simulink model "elevator"  (R2026a)
settings: Solver=VariableStepAuto  StopTime=inf
(part 2 of 2)

== stateflow chart elevator/Chart ==
  state moveup
    entry:
    movedirection=1;
    doorstatus=0;
  state movedown
    entry:
    movedirection=-1;
    doorstatus=0;
  state idle
    entry:
    movedirection=0;
    doorstatus=0;
    during:
    if(floor1==1)
    requestedfloor=0;
    end
    if(floor2==1)
    requestedfloor=1;
    end
    if(floor3==1)
    requestedfloor=2;
    end
  state door_open
    entry:
    movedirection=0;
    doorstatus=1;
  idle -> movedown [order 1] : [requestedfloor<currentfloor]
  (default) -> idle
  movedown -> door_open [order 1] : after(3,sec)[currentfloor==requestedfloor]
  movedown -> movedown [order 2] : after(3,sec)[currentfloor>requestedfloor]{currentfloor=currentfloor-1 }
  idle -> moveup [order 2] : [requestedfloor>currentfloor]
  moveup -> door_open [order 1] : after(3,sec)[currentfloor==requestedfloor]
  moveup -> moveup [order 2] : after(3,sec)[currentfloor<requestedfloor]{currentfloor=currentfloor+1;}
  door_open -> idle : after(5,sec)
  data: movedirection output double =1; doorstatus output double =0; currentfloor output int32 =1; requestedfloor local double =1; floor2 input; floor3 input; floor1 input
